simulink model "Plant_RRSim"  (R2025b)
settings: Solver=FixedStepAuto  StartTime=0.0  StopTime=1000  FixedStep=.01  RelTol=1e-3
values from neighbouring files (symbols this model uses):
  initialVehicleVelocity = 15.6    [LoadDrivingScenario.m]
libraries: autolibshared x1, simulink_extras x1
settings Model: Creator=Jacob  LastModifiedBy=Sam Ball
settings RTWCC: GPUComputeCapability=3.5

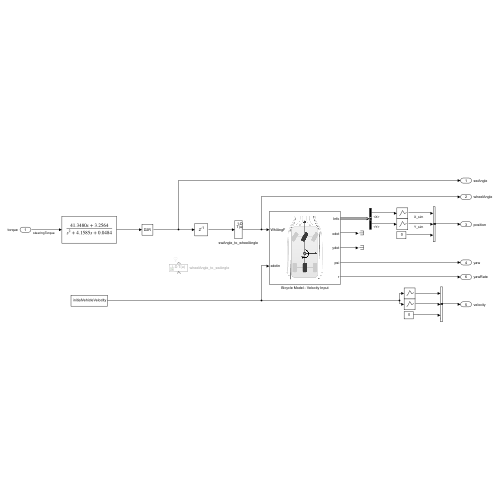
[thumbnail: Simulink's stored preview of the top-level diagram]
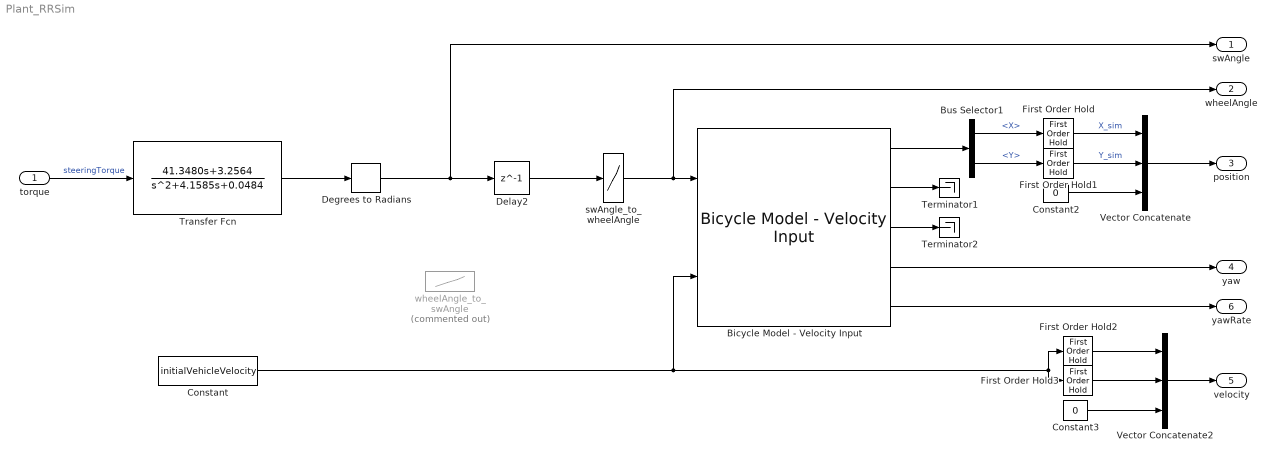
== system Plant_RRSim ==
  torque : Inport
  Bicycle Model - Velocity Input : autolibshared/Bicycle Model - Velocity Input  trackMode=Single (bicycle)  inputMode=External longitudinal velocity  frontSteerMode=on  rearSteerMode=off  windMode=off  muMode=off  extFMode=off  extMMode=off  aMode=3  NF=2  NR=2  m=2765.4  a=1.507  b=1.587  h=0.182  X_o=0  xdot_o=0  CalphaMode=off  sigmaMode=on  w=[1.4,1.4]  Cy_f=12e3  Cy_r=11e3  sigma_f=.1  sigma_r=.1  alpha_f_brk=[-.1 .1]  Cy_f_data=[-9e3 9e3]  alpha_r_brk=[-.1 .1]  Cy_r_data=[-9e3 9e3]  Y_o=0  ydot_o=0  Izz=4000  psi_o=0*pi/180  r_o=0  Af=2  Cd=.3  Cl=.1  Cpm=.1  beta_w=[0 0.01:0.01:0.3]  Cs=[0 0.01:0.01:0.3]  Cym=[0 1e-6:0.01:0.3]  Pabs=101325  Tair=273  g=9.81  mu=1  xdot_tol=.01  Fznom=5000  Fxtire_sat=1e6  Fytire_sat=1e6  longOff=888.7  latOff=-143.6  vertOff=0
      settings: LibrarySourceBlock=drivingscenarioandsensors/Bicycle Model - Velocity Input
  Bus Selector1 : BusSelector  OutputSignals=InertFrm.Cg.Disp.X,InertFrm.Cg.Disp.Y
  Constant : Constant  Value=initialVehicleVelocity
  Constant2 : Constant  Value=0
  Constant3 : Constant  Value=0
  Degrees to Radians : simulink_extras/Transformations/Degrees to Radians
  Delay2 : Delay  DelayLength=1
  First Order Hold{,1..3} (4 alike) : FirstOrderHold  ErrorTolerance=inf  AllowContinuousInput=on
  Terminator1 : Terminator
  Terminator2 : Terminator
  Transfer Fcn : TransferFcn  Numerator=[41.3480 3.2564]  Denominator=[1 4.1585 0.0484]
  Vector Concatenate : Concatenate  NumInputs=3  Mode=Multidimensional array  ConcatenateDimension=2
  Vector Concatenate2 : Concatenate  NumInputs=3  Mode=Multidimensional array  ConcatenateDimension=2
  swAngle_to_wheelAngle : Lookup_n-D  NumberOfTableDimensions=1  BreakpointsForDimension1=[-10.89089966;-10.16600037;-9.441100121;-8.716199875;-7.991300106;-7.26639986;-6.541500092;-5.816599846;-5.091700077;-4.366799831;-3.641900063;-2.917000055;-2.192100048;-1.467200041;-0.742299974;-0.0175;0.0175;0.742299974;1.467200041;2.192100048;2.917000055;3.641900063;4.366799831;5.091700077;5.816599846;6.541500092;7.26639986;7.991300106;8.716199875;9.441100121;10.16600037;10.89089966]  Table=[-0.636900008;-0.589100003;-0.539099991;-0.490500003;-0.44659999;-0.404900014;-0.361499995;-0.317299992;-0.27610001;-0.237499997;-0.197899997;-0.156399995;-0.1162;-0.078699999;-0.041099999;-0.001;0.001;0.041200001;0.079099998;0.116499998;0.156399995;0.197999999;0.237900004;0.276499987;0.317400008;0.361499995;0.405299991;0.447100013;0.490700006;0.539099991;0.589399993;0.637499988]  InternalRulePriority=Speed  RndMeth=Simplest
  wheelAngle_to_swAngle : Lookup_n-D  Commented=on  NumberOfTableDimensions=1  BreakpointsForDimension1=[-0.636900008;-0.589100003;-0.539099991;-0.490500003;-0.44659999;-0.404900014;-0.361499995;-0.317299992;-0.27610001;-0.237499997;-0.197899997;-0.156399995;-0.1162;-0.078699999;-0.041099999;-0.001;0.001;0.041200001;0.079099998;0.116499998;0.156399995;0.197999999;0.237900004;0.276499987;0.317400008;0.361499995;0.405299991;0.447100013;0.490700006;0.539099991;0.589399993;0.637499988]  Table=[-10.89089966;-10.16600037;-9.441100121;-8.716199875;-7.991300106;-7.26639986;-6.541500092;-5.816599846;-5.091700077;-4.366799831;-3.641900063;-2.917000055;-2.192100048;-1.467200041;-0.742299974;-0.0175;0.0175;0.742299974;1.467200041;2.192100048;2.917000055;3.641900063;4.366799831;5.091700077;5.816599846;6.541500092;7.26639986;7.991300106;8.716199875;9.441100121;10.16600037;10.89089966]  InternalRulePriority=Speed  RndMeth=Simplest
  swAngle : Outport
  wheelAngle : Outport  Port=2
  position : Outport  Port=3
  yaw : Outport  Port=4
  velocity : Outport  Port=5
  yawRate : Outport  Port=6
  wires:
  First Order Hold1/1 -> Vector Concatenate/2  "Y_sim"
  Delay2/1 -> swAngle_to_wheelAngle/1
  First Order Hold/1 -> Vector Concatenate/1  "X_sim"
  Bicycle Model - Velocity Input/1 -> Bus Selector1/1
  Bus Selector1/2 -> First Order Hold1/1  "<Y>"
  Constant3/1 -> Vector Concatenate2/3
  Bus Selector1/1 -> First Order Hold/1  "<X>"
  Vector Concatenate2/1 -> velocity/1
  Constant2/1 -> Vector Concatenate/3
  Bicycle Model - Velocity Input/5 -> yawRate/1
  Vector Concatenate/1 -> position/1
  First Order Hold2/1 -> Vector Concatenate2/1
  Bicycle Model - Velocity Input/4 -> yaw/1
  Bicycle Model - Velocity Input/3 -> Terminator2/1
  First Order Hold3/1 -> Vector Concatenate2/2
  Bicycle Model - Velocity Input/2 -> Terminator1/1
  Constant/1 -> First Order Hold3/1, First Order Hold2/1, Bicycle Model - Velocity Input/2
  swAngle_to_wheelAngle/1 -> wheelAngle/1, Bicycle Model - Velocity Input/1
  torque/1 -> Transfer Fcn/1  "steeringTorque"
  Transfer Fcn/1 -> Degrees to Radians/1
  Degrees to Radians/1 -> Delay2/1, swAngle/1
